simulink model "EMEA_Controls_States"  (Simulink 8.7)
settings: Solver=FixedStepDiscrete  StartTime=0.0  StopTime=10.0  FixedStep=0.1  RelTol=1e-3
settings Model: Creator=aliebel  LastModifiedBy=aliebel
settings SolverCC: AutoInsertRateTranBlk=on
settings DataIOCC: SaveFormat=Dataset
settings DebuggingCC: UnderspecifiedInitializationDetection=Simplified  MergeDetectMultiDrivingBlocksExec=error  AllowSymbolicDim=off
settings HardwareCC: ProdBitPerPointer=64  ProdLargestAtomicFloat=Float  ProdIntDivRoundTo=Zero  ProdEndianess=LittleEndian  ProdWordSize=64  ProdHWDeviceType=Intel->x86-64 (Windows64)
settings ModelReferenceCC: PropagateSignalLabelsOutOfModel=on
settings ConfigComp: CovSFcnEnable=off

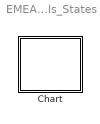
== system EMEA_Controls_States ==
  Chart : Stateflow chart  TreatAsAtomicUnit=on

== stateflow chart Chart ==
  state OptionA
    state StateA3
      % Aux Disabled
      % Offset Enabled
      % Display __:__
    state StateG1
      % Aux Enabled
      % Offset Enabled
      % Display A4:A1
    state StateA
      % Aux Disabled
      % Offset Enabled
      % Display OF:__
    state StateB1
      % Aux Enabled
      % Offset Enabled
      % Display OF:A1
    state StateB
      % Aux Enabled
      % Offset Enabled
      % Display OF:A1
    state StateC3
      % Aux Disabled
      % OffsetEnabled
      % Display __:OF
    state StateC4
      % Aux Enabled
      % Offset Enabled
      % Display OF:A4
    state StateC2
      % Aux Disabled
      % OffsetEnabled
      % Display __:OF
      % Flash Aux Button **
    note: ** Only flash aux lights if not coming from key on
        | or if coming from an intentional aux disable
    state StateA1
      % Aux Disabled
      % Offset Enabled
      % Display OF:__
    state StateC
      % Aux Enabled
      % Offset Enabled
      % Display A2:A1
    state StateD1
      % Aux Enabled
      % Offset Enabled
      % Display A4:OF
    state StateD2
      % Aux Enabled
      % Offset Enabled
      % Display A4:OF
    state KeyOff
    state KeyOff1
    state StateA2
      % Aux Disabled
      % Offset Enabled
      % Display OF:__
      % Flash Aux Button**
    note: Right Mode
    note: Left Mode
    note: Any pot out of neutral will not allow state change
        | Also need to consider what happens if console is up or fault conditions
    state KeyOff2
    (default) -> KeyOff2 [order 3]
    (default) -> OptionA.KeyOff [order 1]
    (default) -> KeyOff1 [order 2]
    KeyOff2 -> (junction 65) : [Key On]
    OptionA.KeyOff -> OptionA.StateA3 : [Key On]
    KeyOff1 -> (junction 66) : [Key On]
    StateC4 -> StateA2 [order 2] : [!enable_aux]
        | % no pot checks
        | % single beep (aux button)
    OptionA.StateC -> OptionA.StateA [order 2] : [!enable_aux]
        | % no pot checks
        | % single beep (aux button)
    (junction 65) -> StateC3 [order 2] : [OffsetRight]
    (junction 66) -> StateC2 [order 2] : [OffsetRight]
    (junction 65) -> StateA2 [order 1] : [OffsetLeft]
    (junction 66) -> StateA1 [order 1] : [OffsetLeft]
    OptionA.StateA3 -> OptionA.StateA : %check left pot
    OptionA.StateB1 -> StateC4 [order 2] : [changeRightMode]
        | %check right pot
        | %single beep
    StateA2 -> OptionA.StateB1 [order 1] : [enable_aux]
        | %aux enable checks right pot
        | %no check for left pot
        | %single beep (aux button)
    StateA2 -> StateA2 [order 3] : [changeRightMode]
        | % 3 beeps
    OptionA.StateB -> OptionA.StateC [order 1] : [changeLeftMode]
        | %check left pot
        | %double beep
    OptionA.StateA -> OptionA.StateB [order 1] : [enable_aux]
        | %aux enable checks right pot
        | %no check for left pot
        | %single beep (aux button)
    OptionA.StateA -> OptionA.StateA [order 2] : [changeLeftMode]
        | % 3 beeps
    StateD1 -> StateA1 [order 2] : [OffsetLeft]
        | % check left pot
        | % medium beep
    OptionA.StateB1 -> StateA2 [order 3] : [!enable_aux]
        | % no pot checks
        | % single beep (aux button)
    StateC4 -> OptionA.StateB1 [order 1] : [changeRightMode]
        | %check right pot
        | %single beep
    OptionA.StateB -> OptionA.StateA [order 2] : [!enable_aux]
        | % no pot checks
        | % single beep (aux button)
    OptionA.StateC -> OptionA.StateB [order 1] : [changeLeftMode]
        | %check left pot
        | %single beep
    StateC3 -> StateA2 [order 2] : [OffsetLeft]
        | % check left pot
        | % medium beep
    StateA2 -> StateC3 [order 2] : [OffsetRight]
        | % check right pot
        | % Medium Beep
    (junction 72) -> StateA2
    OptionA.StateB1 -> (junction 68) [order 1] : [OffsetRight]
        | % check right pot
        | % Medium Beep
    StateC4 -> (junction 69) [order 3] : [OffsetRight]
        | % check right pot
        | % Medium Beep
    StateC2 -> StateA1 [order 2] : [OffsetLeft]
        | % check left pot
        | % medium beep
    StateA1 -> StateC2 : [OffsetRight]
        | % check right pot
        | % Medium Beep
    (junction 68) -> (junction 67)
    (junction 69) -> (junction 68)
    (junction 67) -> StateC3
    (junction 70) -> (junction 71)
    (junction 71) -> (junction 72)
    StateG1 -> (junction 70) [order 2] : [OffsetLeft]
        | % check left pot
        | % medium beep
    StateD2 -> (junction 71) [order 1] : [OffsetLeft]
        | % check left pot
        | % medium beep
    StateD2 -> StateG1 [order 3] : [changeRightMode]
        | %check right pot
        | %single beep
    StateC3 -> StateC3 [order 3] : [changeRightMode]
        | % 3 beeps
    StateC3 -> StateD2 [order 1] : [enable_aux]
        | % aux enable checks right pot
        | % check left pot
        | % single beep (aux button)
    StateC2 -> StateD1 [order 1] : [enable_aux]
        | % aux enable checks right pot
        | % check left pot
        | % single beep (aux button)
    StateD2 -> StateC3 [order 2] : [!enable_aux]
        | % no pot checks
        | % single beep (aux button)
    StateG1 -> StateD2 [order 1] : [changeRightMode]
        | %check right pot
        | %single beep
    StateD1 -> StateC2 [order 1] : [!enable_aux]
        | % no pot checks
        | % single beep (aux button)
    StateG1 -> StateC3 [order 3] : [!enable_aux]
        | % no pot checks
        | % single beep (aux button)
  state OptionC
    note: Any pot out of neutral will not allow state change
        | Also need to consider what happens if console is up or fault conditions
    state KeyOff
    state StateA3
      % Aux Disabled
      % Offset Disabled
      % Display __:__
      % No Aux button flash
    state OffsetRight
      state StateC
        % Aux Disabled
        % OffsetEnabled
        % Display __:OF
      state Aux_Enabled
        state StateD
          % Aux Enabled
          % Offset Enabled
          % Display A4:OF
          % No Aux button flash
        state StateG
          % Aux Enabled
          % Offset Enabled
          % Display A4:A1
        state StateB3
          % Aux Enabled
          % Offset Enabled
          % Display A2:A1
        OptionC.OffsetRight.Aux_Enabled.StateD -> OptionC.OffsetRight.Aux_Enabled.StateG [order 1] : [changeRightMode]
            | %check right pot
            | %double beep
        OptionC.OffsetRight.Aux_Enabled.StateG -> OptionC.OffsetRight.Aux_Enabled.StateD [order 2] : [changeRightMode]
            | %check right pot
            | %single beep
        OptionC.OffsetRight.Aux_Enabled.StateD -> OptionC.OffsetRight.Aux_Enabled.StateD [order 2] : [changeLeftMode]
            | % 3 beeps
        OptionC.OffsetRight.Aux_Enabled.StateG -> StateB3 [order 1] : [changeLeftMode]
            | %check left pot
            | %double beep
        StateB3 -> OptionC.OffsetRight.Aux_Enabled.StateG [order 1] : [changeLeftMode]
            | %check left pot
            | %single beep
        StateB3 -> StateB3 [order 2] : [changeLeftMode]
            | % 3 beeps
      OptionC.OffsetRight.StateC -> OptionC.OffsetRight.StateC [order 2] : [changeRightMode...
          | || changeLeftMode]
          | % 3 beeps
      OptionC.OffsetRight.StateC -> OptionC.OffsetRight.Aux_Enabled [order 1] : [enable_aux]
          | % aux enable checks right pot
          | % check left pot
          | % single beep (aux button)
      OptionC.OffsetRight.Aux_Enabled -> OptionC.OffsetRight.StateC : [!enable_aux]
          | % no pot checks
          | % single beep (aux button)
    state OffsetLeft
      state StateA
        % Aux Disabled
        % Offset Enabled
        % Display OF:__
      state Aux_Enabled
        state StateB
          % Aux Enabled
          % Offset Enabled
          % Display OF:A1
          % No Aux button flash
        state StateC1
          % Aux Enabled
          % Offset Enabled
          % Display OF:A4
        state StateB1
          % Aux Enabled
          % Offset Enabled
          % Display A2:A1
        state StateB2
          % Aux Enabled
          % Offset Enabled
          % Display A2:A4
        (default) -> OptionC.OffsetLeft.Aux_Enabled.StateB
        OptionC.OffsetLeft.Aux_Enabled.StateB -> OptionC.OffsetLeft.Aux_Enabled.StateC1 [order 1] : [changeRightMode]
            | %check right pot
            | %double beep
        OptionC.OffsetLeft.Aux_Enabled.StateC1 -> OptionC.OffsetLeft.Aux_Enabled.StateB [order 2] : [changeRightMode]
            | %check right pot
            | %single beep
        OptionC.OffsetLeft.Aux_Enabled.StateC1 -> StateB2 [order 1] : [changeLeftMode]
            | %check left pot
            | %double beep
        StateB2 -> OptionC.OffsetLeft.Aux_Enabled.StateC1 [order 1] : [changeLeftMode]
            | %check left pot
            | %single beep
        OptionC.OffsetLeft.Aux_Enabled.StateB -> OptionC.OffsetLeft.Aux_Enabled.StateB1 [order 2] : [changeLeftMode]
            | %check left pot
            | %double beep
        OptionC.OffsetLeft.Aux_Enabled.StateB1 -> OptionC.OffsetLeft.Aux_Enabled.StateB [order 1] : [changeLeftMode]
            | %check left pot
            | %single beep
        OptionC.OffsetLeft.Aux_Enabled.StateB1 -> StateB2 [order 2] : [changeRightMode]
            | %check right pot
            | %double beep
        StateB2 -> OptionC.OffsetLeft.Aux_Enabled.StateB1 [order 2] : [changeRightMode]
            | %check right pot
            | %single beep
      OptionC.OffsetLeft.StateA -> OptionC.OffsetLeft.StateA [order 2] : [changeRightMode...
          | || changeLeftMode]
          | % 3 beeps
      OptionC.OffsetLeft.StateA -> OptionC.OffsetLeft.Aux_Enabled [order 1] : [enable_aux]
          | %aux enable checks right pot
          | %no check for left pot
          | %single beep (aux button)
      OptionC.OffsetLeft.Aux_Enabled -> OptionC.OffsetLeft.StateA : [!enable_aux]
          | % no pot checks
          | % single beep (aux button)
    (default) -> OptionC.KeyOff
    OptionC.KeyOff -> OptionC.StateA3 : [Key On]
    OptionC.StateA3 -> (junction 119)
    (junction 119) -> OptionC.OffsetRight [order 2] : [OffsetRight]
        | %check right pot
    (junction 119) -> OptionC.OffsetLeft.StateA [order 1] : [OffsetLeft]
        | %check left pot
    OptionC.OffsetRight -> OptionC.OffsetLeft : [OffsetLeft]
        | % check left pot
        | % medium beep
        | % Flash Aux Button
    OptionC.OffsetLeft -> OptionC.OffsetRight : [OffsetRight]
        | % check right pot
        | % Medium Beep
        | % Flash Aux Button
  state OptionB
    state KeyOff
    state OffsetRight
      state StateC
        % Aux Disabled
        % OffsetEnabled
        % Display __:OF
      state StateD
        % Aux Enabled
        % Offset Enabled
        % Display A4:OF
        % No Aux button flash
      state StateG
        % Aux Enabled
        % Offset Enabled
        % Display A4:A1
      OptionB.OffsetRight.StateD -> OptionB.OffsetRight.StateG [order 2] : [changeRightMode]
          | %check right pot
          | %double beep
      OptionB.OffsetRight.StateC -> OptionB.OffsetRight.StateC [order 2] : [changeRightMode]
          | % 3 beeps
      OptionB.OffsetRight.StateC -> OptionB.OffsetRight.StateD [order 1] : [enable_aux]
          | % aux enable checks right pot
          | % check left pot
          | % single beep (aux button)
      OptionB.OffsetRight.StateD -> OptionB.OffsetRight.StateC [order 1] : [!enable_aux]
          | % no pot checks
          | % single beep (aux button)
      OptionB.OffsetRight.StateG -> OptionB.OffsetRight.StateD [order 2] : [changeRightMode]
          | %check right pot
          | %single beep
      OptionB.OffsetRight.StateG -> OptionB.OffsetRight.StateC [order 1] : [!enable_aux]
          | % no pot checks
          | % single beep (aux button)
    state OffsetLeft
      state StateB
        % Aux Enabled
        % Offset Enabled
        % Display OF:A1
        % No Aux button flash
      state StateA
        % Aux Disabled
        % Offset Enabled
        % Display OF:__
      state StateC1
        % Aux Enabled
        % Offset Enabled
        % Display OF:A4
      OptionB.OffsetLeft.StateB -> OptionB.OffsetLeft.StateC1 [order 1] : [changeRightMode]
          | %check right pot
          | %double beep
      OptionB.OffsetLeft.StateA -> OptionB.OffsetLeft.StateB [order 1] : [enable_aux]
          | %aux enable checks right pot
          | %no check for left pot
          | %single beep (aux button)
      OptionB.OffsetLeft.StateA -> OptionB.OffsetLeft.StateA [order 2] : [changeRightMode]
          | % 3 beeps
      OptionB.OffsetLeft.StateB -> OptionB.OffsetLeft.StateA [order 2] : [!enable_aux]
          | % no pot checks
          | % single beep (aux button)
      OptionB.OffsetLeft.StateC1 -> OptionB.OffsetLeft.StateB [order 1] : [changeRightMode]
          | %check right pot
          | %single beep
      OptionB.OffsetLeft.StateC1 -> OptionB.OffsetLeft.StateA [order 2] : [!enable_aux]
          | % no pot checks
          | % single beep (aux button)
    state StateA3
      % Aux Disabled
      % Offset Disabled
      % Display __:__
      % No Aux button flash
    note: Any pot out of neutral will not allow state change
        | Also need to consider what happens if console is up or fault conditions
    (default) -> OptionB.KeyOff
    OptionB.KeyOff -> OptionB.StateA3 : [Key On]
    OptionB.StateA3 -> (junction 133)
    (junction 133) -> OptionB.OffsetRight [order 2] : [OffsetRight]
        | %check right pot
    (junction 133) -> OptionB.OffsetLeft.StateA [order 1] : [OffsetLeft]
        | %check left pot
    OptionB.OffsetRight -> OptionB.OffsetLeft : [OffsetLeft]
        | % check left pot
        | % medium beep
        | % Flash Aux Button
    OptionB.OffsetLeft -> OptionB.OffsetRight : [OffsetRight]
        | % check right pot
        | % Medium Beep
        | % Flash Aux Button
